simulink model "PendulumModel_wIntegralControl"  (R2018b)
settings: Solver=ode45  StartTime=0.0  StopTime=tend  FixedStep=1e-3  MaxStep=0.1  RelTol=1e-3  EnableMultiTasking=on
values from neighbouring files (symbols this model uses):
  D = [0]    [Pendulum_Controller.m]    (also in Robot_Grasper.m)
  g = 9.81    [Pendulum_Controller.m]
  J = m*L/3    (= 0.166666666667)    [Pendulum_Controller.m]
  K = Kall(1:(end-1))    [Pendulum_Controller.m]
  Ki = -Kall(end)    [Pendulum_Controller.m]    (also in Robot_Grasper.m = acker(Ai, Bi, [desiredPoles' -400]))
  L = 1    [Pendulum_Controller.m]    (also in Robot_Grasper.m = acker( A', C', desiredObsPoles)')
  m = 0.5    [Pendulum_Controller.m]    (also in Robot_Grasper.m = 0.155)
  theta_0 = 175 * [pi/180]    [Pendulum_Controller.m]
  theta_setPoint = 180 *pi/180    (= 3.14159265359)    [Pendulum_Controller.m]
settings Model: Creator=pjseiler  LastModifiedBy=holdentranquillo
settings SolverCC: AlgebraicLoopSolver=LineSearch
settings DataIOCC: SaveFormat=Array
settings OptimizationCC: ExpressionDepthLimit=2147483647  LifeSpan=inf
settings DebuggingCC: UnderspecifiedInitializationDetection=Classic  MergeDetectMultiDrivingBlocksExec=none  SolverPrmCheckMsg=warning  MultiTaskDSMMsg=warning  MultiTaskCondExecSysMsg=none  FcnCallInpInsideContextMsg=warning  StateNameClashWarn=warning  LibraryContextMissingDiagnostic=none  SFUnexpectedBacktrackingDiag=warning  SFNoUnconditionalDefaultTransitionDiag=warning  SFExecutionAtInitializationDiag=none
settings HardwareCC: ProdBitPerPointer=32  ProdBitPerSizeT=32  ProdBitPerPtrDiffT=32  ProdLargestAtomicFloat=None  ProdIntDivRoundTo=Undefined  ProdEndianess=Unspecified  ProdWordSize=32  ProdHWDeviceType=32-bit Generic
settings ModelReferenceCC: PropagateSignalLabelsOutOfModel=off
settings SFSimCC: SimUseLocalCustomCode=off
settings RTWCC: RTWUseLocalCustomCode=off
settings CodeAppCC: StateflowObjectComments=on
settings GRTTargetCC: TargetLangStandard=C89/C90 (ANSI)  GeneratePreprocessorConditionals=Disable all  CombineOutputUpdateFcns=off  GRTInterface=on
settings ConfigComp: CovMetricSettings=dw  CovHtmlReporting=on  CovSaveCumulativeToWorkspaceVar=on  CovSaveSingleToWorkspaceVar=on  CovExternalEMLEnable=off  CovSFcnEnable=off

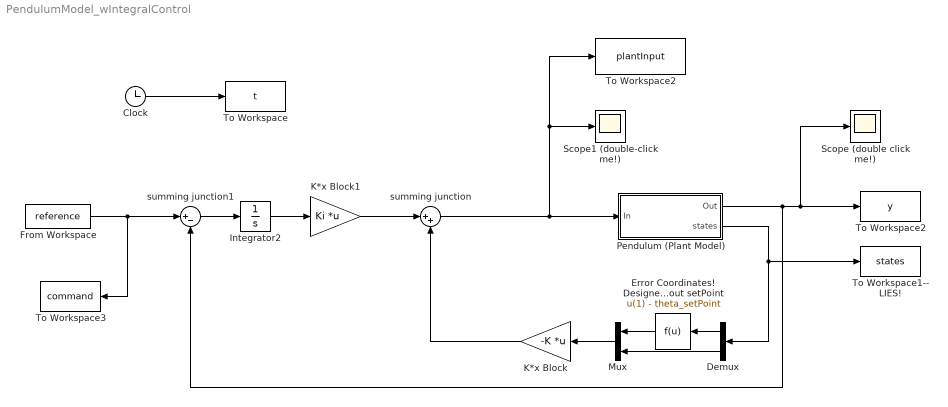
== system PendulumModel_wIntegralControl ==
  Clock : Clock
  Demux : Demux  Outputs=2
  Error Coordinates! Designed K about setPoint : Fcn  Expr=u(1) - theta_setPoint
  From Workspace : FromWorkspace  VariableName=reference  SampleTime=0
  Integrator2 : Integrator
  K*x Block : Gain  Gain=-K  Multiplication=Matrix(K*u)
  K*x Block1 : Gain  Gain=Ki  Multiplication=Matrix(K*u)
  Mux : Mux  Inputs=2
  "Pendulum (Plant Model) " : Subsystem
  Scope (double click me!) : Scope
  Scope1 (double-click me!) : Scope
  To Workspace : ToWorkspace  VariableName=t  SampleTime=-1
  To Workspace1-- LIES! : ToWorkspace  VariableName=states  SampleTime=-1
  To Workspace2 : ToWorkspace  VariableName=y  SampleTime=-1
  "To Workspace2 " : ToWorkspace  VariableName=plantInput  SampleTime=-1
  To Workspace3 : ToWorkspace  VariableName=command  SampleTime=-1
  summing junction : Sum  Inputs=|++
  summing junction1 : Sum  Inputs=|+-
  wires:
  Clock/1 -> To Workspace/1
  "Pendulum (Plant Model) "/1(Out) -> To Workspace2/1, Scope (double click me!)/1, summing junction1/2
  "Pendulum (Plant Model) "/2(states) -> Demux/1, To Workspace1-- LIES!/1
  K*x Block/1 -> summing junction/2
  Mux/1 -> K*x Block/1
  Demux/1 -> Error Coordinates! Designed K about setPoint/1
  Error Coordinates! Designed K about setPoint/1 -> Mux/1
  Demux/2 -> Mux/2
  From Workspace/1 -> summing junction1/1, To Workspace3/1
  summing junction/1 -> "To Workspace2 "/1, Scope1 (double-click me!)/1, "Pendulum (Plant Model) "/1(In)
  K*x Block1/1 -> summing junction/1
  Integrator2/1 -> K*x Block1/1
  summing junction1/1 -> Integrator2/1

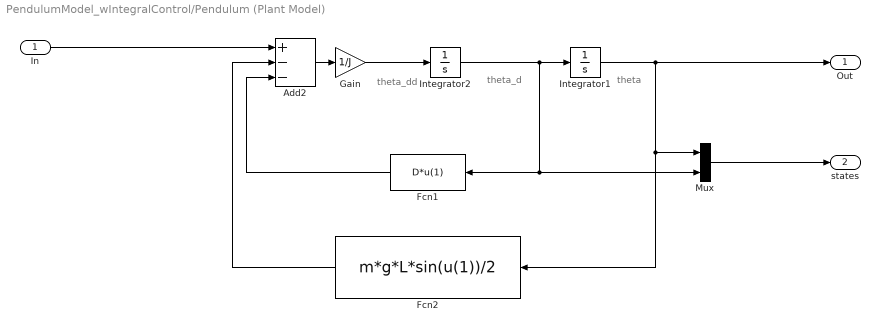
== system PendulumModel_wIntegralControl/Pendulum (Plant Model)  ==
  note: theta_dd
  note: theta_d
  note: theta
  In : Inport
  Add2 : Sum  Inputs=+--
  Fcn1 : Fcn  Expr=D*u(1)
  Fcn2 : Fcn  Expr=m*g*L*sin(u(1))/2
  Gain : Gain  Gain=1/J
  Integrator1 : Integrator  InitialCondition=theta_0
  Integrator2 : Integrator
  Mux : Mux  Inputs=2
  Out : Outport
  states : Outport  Port=2
  wires:
  Integrator2/1 -> Mux/2, Fcn1/1, Integrator1/1
  Integrator1/1 -> Mux/1, Fcn2/1, Out/1
  Add2/1 -> Gain/1
  Fcn1/1 -> Add2/3
  Fcn2/1 -> Add2/2
  In/1 -> Add2/1
  Mux/1 -> states/1
  Gain/1 -> Integrator2/1
